simulink model "sys_1_statespace"  (R2017a)
settings: Solver=VariableStepAuto  StartTime=0.0  StopTime=25  FixedStep=0.02  RelTol=1e-3
values from neighbouring files (symbols this model uses):
  A = [0 1 0 0;-k/j2 -b/j2 k/j2 b/j2;0 0 0 01;k/j1 b/j1 -k/j1 -b/j1]    [sys1.m]
  A3 = [0 1 0 0;-k/j2 -b/j2 k/j2 b/j2;0 0 0 01;k/j1 b/j1 -k/j1 -b/j1]    [sys1.m]
  B = [b -b;-b b]    [dynamic_using_Nemark_controller.m]    (also in sys1.m = [0;0;0;1/j1])
  B3 = [0;0;0;1/j1]    [sys1.m]
  C = [1 0 0 0]    [sys1.m]
  C3 = [0 0 1 0;1 0 0 0]    [sys1.m]
  D = zeros(1,1)    [sys1.m]
  D3 = zeros(2,1)    [sys1.m]
undefined symbols (not defined in the file or in its folder): Ad, Bd, Cd, Dd
libraries: simulink x10
settings Model: Creator=ASUS  LastModifiedBy=ASUS

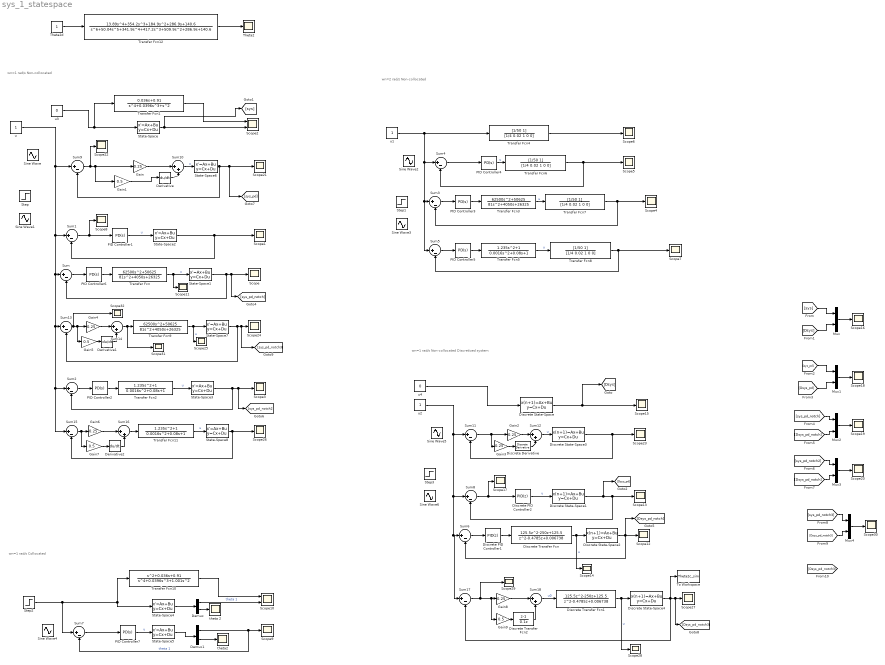
== system sys_1_statespace ==
  note: wn=1 rad/s Non-collocated
  note: wn=2 rad/s Non-collocated
  note: wn=1 rad/s Collocated
  note: wn=1 rad/s Non-collocated
      | Discretized system
  Demux : Demux  Outputs=2
  Demux1 : Demux  Outputs=2
  Derivative : Derivative
  Derivative1 : Derivative
  Derivative2 : Derivative
  Discrete Transfer Fcn : DiscreteTransferFcn  Numerator=[125.5 -250 125.5]  Denominator=[1 -0.4785 0.006738]  SampleTime=0.1
  Discrete Transfer Fcn1 : DiscreteTransferFcn  Numerator=[125.5 -250 125.5]  Denominator=[1 -0.4785 0.006738]  SampleTime=0.1
  Discrete Transfer Fcn2 : DiscreteTransferFcn  Numerator=[1 -1]  Denominator=[0.1 0]  SampleTime=0.1
  Discrete Derivative : simulink/Discrete/Discrete Derivative  gainval=1.0  ICPrevScaledInput=0.0  OutMin=[]  OutMax=[]  OutDataType=fixdt(1, 16)  OutScaling=2^-10  DoSatur=off
  Discrete PID Controller1 : simulink/Continuous/PID Controller  Controller=PID  TimeDomain=Discrete-time  SampleTime=0.1  IntegratorMethod=Forward Euler  FilterMethod=Forward Euler  Form=Parallel  UseFilter=on  ControllerParametersSource=internal  P=0.25  I=0  D=0.5  N=1  InitialConditionSource=internal  InitialConditionForIntegrator=0  InitialConditionForFilter=0  ExternalReset=none  LimitOutput=off  UpperSaturationLimit=inf  LowerSaturationLimit=-inf  LinearizeAsGain=off  AntiWindupMode=none  Kb=1  TrackingMode=off  Kt=1  PParamMin=[]  PParamMax=[]  IParamMin=[]  IParamMax=[]  DParamMin=[]  DParamMax=[]  NParamMin=[]  NParamMax=[]  KbParamMin=[]  KbParamMax=[]  KtParamMin=[]  KtParamMax=[]  POutMin=[]  POutMax=[]  IOutMin=[]  IOutMax=[]  DOutMin=[]  DOutMax=[]  NOutMin=[]  NOutMax=[]  KbOutMin=[]  KbOutMax=[]  KtOutMin=[]  KtOutMax=[]  IntegratorOutMin=[]  IntegratorOutMax=[]  FilterOutMin=[]  FilterOutMax=[]  SumOutMin=[]  SumOutMax=[]  SumI1OutMin=[]  SumI1OutMax=[]  SumI2OutMin=[]  SumI2OutMax=[]  SumI3OutMin=[]  SumI3OutMax=[]  SumDOutMin=[]  SumDOutMax=[]  SaturationOutMin=[]  SaturationOutMax=[]  IntegratorContinuousStateAttributes=''  IntegratorStateMustResolveToSignalObject=off  IntegratorRTWStateStorageClass=Auto  FilterContinuousStateAttributes=''  FilterStateMustResolveToSignalObject=off  FilterRTWStateStorageClass=Auto  DifferentiatorICPrevScaledInput=0  DifferentiatorOutMin=[]  DifferentiatorOutMax=[]  InitialConditionSetting=State (most efficient)
  Discrete PID Controller2 : simulink/Continuous/PID Controller  Controller=PID  TimeDomain=Discrete-time  SampleTime=0.10  IntegratorMethod=Forward Euler  FilterMethod=Forward Euler  Form=Parallel  UseFilter=on  ControllerParametersSource=internal  P=0.25  I=0  D=0.5  N=1  InitialConditionSource=internal  InitialConditionForIntegrator=0  InitialConditionForFilter=0  ExternalReset=none  LimitOutput=off  UpperSaturationLimit=inf  LowerSaturationLimit=-inf  LinearizeAsGain=off  AntiWindupMode=none  Kb=1  TrackingMode=off  Kt=1  PParamMin=[]  PParamMax=[]  IParamMin=[]  IParamMax=[]  DParamMin=[]  DParamMax=[]  NParamMin=[]  NParamMax=[]  KbParamMin=[]  KbParamMax=[]  KtParamMin=[]  KtParamMax=[]  POutMin=[]  POutMax=[]  IOutMin=[]  IOutMax=[]  DOutMin=[]  DOutMax=[]  NOutMin=[]  NOutMax=[]  KbOutMin=[]  KbOutMax=[]  KtOutMin=[]  KtOutMax=[]  IntegratorOutMin=[]  IntegratorOutMax=[]  FilterOutMin=[]  FilterOutMax=[]  SumOutMin=[]  SumOutMax=[]  SumI1OutMin=[]  SumI1OutMax=[]  SumI2OutMin=[]  SumI2OutMax=[]  SumI3OutMin=[]  SumI3OutMax=[]  SumDOutMin=[]  SumDOutMax=[]  SaturationOutMin=[]  SaturationOutMax=[]  IntegratorContinuousStateAttributes=''  IntegratorStateMustResolveToSignalObject=off  IntegratorRTWStateStorageClass=Auto  FilterContinuousStateAttributes=''  FilterStateMustResolveToSignalObject=off  FilterRTWStateStorageClass=Auto  DifferentiatorICPrevScaledInput=0  DifferentiatorOutMin=[]  DifferentiatorOutMax=[]  InitialConditionSetting=State (most efficient)
  Discrete State-Space{,1..4} (5 alike) : DiscreteStateSpace  A=Ad  B=Bd  C=Cd  D=Dd  X0=[0.2 0 0 0]  SampleTime=0.1
  Gain{,2..4,6,8} (6 alike) : Gain  Gain=0.25
  Gain{1,5,7,9} (4 alike) : Gain  Gain=0.5
  Mux{,1..4} (5 alike) : Mux  Inputs=2
  PID Controller{1..3,5,7} (5 alike) : simulink/Continuous/PID Controller  Controller=PD  TimeDomain=Continuous-time  SampleTime=-1  IntegratorMethod=Forward Euler  FilterMethod=Forward Euler  Form=Parallel  UseFilter=on  ControllerParametersSource=internal  P=0.25  I=0  D=0.5  N=100  InitialConditionSource=internal  InitialConditionForIntegrator=0  InitialConditionForFilter=0  ExternalReset=none  LimitOutput=off  UpperSaturationLimit=inf  LowerSaturationLimit=-inf  LinearizeAsGain=on  AntiWindupMode=none  Kb=1  TrackingMode=off  Kt=1  PParamMin=[]  PParamMax=[]  IParamMin=[]  IParamMax=[]  DParamMin=[]  DParamMax=[]  NParamMin=[]  NParamMax=[]  KbParamMin=[]  KbParamMax=[]  KtParamMin=[]  KtParamMax=[]  POutMin=[]  POutMax=[]  IOutMin=[]  IOutMax=[]  DOutMin=[]  DOutMax=[]  NOutMin=[]  NOutMax=[]  KbOutMin=[]  KbOutMax=[]  KtOutMin=[]  KtOutMax=[]  IntegratorOutMin=[]  IntegratorOutMax=[]  FilterOutMin=[]  FilterOutMax=[]  SumOutMin=[]  SumOutMax=[]  SumI1OutMin=[]  SumI1OutMax=[]  SumI2OutMin=[]  SumI2OutMax=[]  SumI3OutMin=[]  SumI3OutMax=[]  SumDOutMin=[]  SumDOutMax=[]  SaturationOutMin=[]  SaturationOutMax=[]  IntegratorContinuousStateAttributes=''  IntegratorStateMustResolveToSignalObject=off  IntegratorRTWStateStorageClass=Auto  FilterContinuousStateAttributes=''  FilterStateMustResolveToSignalObject=off  FilterRTWStateStorageClass=Auto  DifferentiatorICPrevScaledInput=0  DifferentiatorOutMin=[]  DifferentiatorOutMax=[]  InitialConditionSetting=State (most efficient)
  PID Controller4 : simulink/Continuous/PID Controller  Controller=PD  TimeDomain=Continuous-time  SampleTime=-1  IntegratorMethod=Forward Euler  FilterMethod=Forward Euler  Form=Parallel  UseFilter=on  ControllerParametersSource=internal  P=0.001  I=0  D=0.03  N=100  InitialConditionSource=internal  InitialConditionForIntegrator=0  InitialConditionForFilter=0  ExternalReset=none  LimitOutput=off  UpperSaturationLimit=inf  LowerSaturationLimit=-inf  LinearizeAsGain=on  AntiWindupMode=none  Kb=1  TrackingMode=off  Kt=1  PParamMin=[]  PParamMax=[]  IParamMin=[]  IParamMax=[]  DParamMin=[]  DParamMax=[]  NParamMin=[]  NParamMax=[]  KbParamMin=[]  KbParamMax=[]  KtParamMin=[]  KtParamMax=[]  POutMin=[]  POutMax=[]  IOutMin=[]  IOutMax=[]  DOutMin=[]  DOutMax=[]  NOutMin=[]  NOutMax=[]  KbOutMin=[]  KbOutMax=[]  KtOutMin=[]  KtOutMax=[]  IntegratorOutMin=[]  IntegratorOutMax=[]  FilterOutMin=[]  FilterOutMax=[]  SumOutMin=[]  SumOutMax=[]  SumI1OutMin=[]  SumI1OutMax=[]  SumI2OutMin=[]  SumI2OutMax=[]  SumI3OutMin=[]  SumI3OutMax=[]  SumDOutMin=[]  SumDOutMax=[]  SaturationOutMin=[]  SaturationOutMax=[]  IntegratorContinuousStateAttributes=''  IntegratorStateMustResolveToSignalObject=off  IntegratorRTWStateStorageClass=Auto  FilterContinuousStateAttributes=''  FilterStateMustResolveToSignalObject=off  FilterRTWStateStorageClass=Auto  DifferentiatorICPrevScaledInput=0  DifferentiatorOutMin=[]  DifferentiatorOutMax=[]  InitialConditionSetting=State (most efficient)
  PID Controller6 : simulink/Continuous/PID Controller  Controller=PD  TimeDomain=Continuous-time  SampleTime=-1  IntegratorMethod=Forward Euler  FilterMethod=Forward Euler  Form=Parallel  UseFilter=on  ControllerParametersSource=internal  P=0.25  I=0  D=0.5  N=1  InitialConditionSource=internal  InitialConditionForIntegrator=0  InitialConditionForFilter=0  ExternalReset=none  LimitOutput=off  UpperSaturationLimit=inf  LowerSaturationLimit=-inf  LinearizeAsGain=on  AntiWindupMode=none  Kb=1  TrackingMode=off  Kt=1  PParamMin=[]  PParamMax=[]  IParamMin=[]  IParamMax=[]  DParamMin=[]  DParamMax=[]  NParamMin=[]  NParamMax=[]  KbParamMin=[]  KbParamMax=[]  KtParamMin=[]  KtParamMax=[]  POutMin=[]  POutMax=[]  IOutMin=[]  IOutMax=[]  DOutMin=[]  DOutMax=[]  NOutMin=[]  NOutMax=[]  KbOutMin=[]  KbOutMax=[]  KtOutMin=[]  KtOutMax=[]  IntegratorOutMin=[]  IntegratorOutMax=[]  FilterOutMin=[]  FilterOutMax=[]  SumOutMin=[]  SumOutMax=[]  SumI1OutMin=[]  SumI1OutMax=[]  SumI2OutMin=[]  SumI2OutMax=[]  SumI3OutMin=[]  SumI3OutMax=[]  SumDOutMin=[]  SumDOutMax=[]  SaturationOutMin=[]  SaturationOutMax=[]  IntegratorContinuousStateAttributes=''  IntegratorStateMustResolveToSignalObject=off  IntegratorRTWStateStorageClass=Auto  FilterContinuousStateAttributes=''  FilterStateMustResolveToSignalObject=off  FilterRTWStateStorageClass=Auto  DifferentiatorICPrevScaledInput=0  DifferentiatorOutMin=[]  DifferentiatorOutMax=[]  InitialConditionSetting=State (most efficient)
  Scope{,1,3..9,11..32} (31 alike) : Scope
  Scope10 : Scope  NumInputPorts=2
  Scope2 : Scope  NumInputPorts=2
  Sine Wave{,2,4..5} (4 alike) : Sin  Frequency=3  SampleTime=0
  Sine Wave1 : Sin  SampleTime=0
  Sine Wave3 : Sin  SampleTime=0
  Sine Wave6 : Sin  SampleTime=0
  State-Space{,1..3,6..8} (7 alike) : StateSpace  A=A  B=B  C=C  D=D  X0=[0.2 0 0 0]
  State-Space4 : StateSpace  A=A3  B=B3  C=C3  D=D3  X0=0
  State-Space5 : StateSpace  A=A3  B=B3  C=C3  D=D3  X0=0
  Step{,1..3} (4 alike) : Step  SampleTime=0
  Sum{,1..9,11,13,15,17} (14 alike) : Sum  Inputs=|+-
  Sum{10,12,14,16,18} (5 alike) : Sum  Inputs=|++
  Theta2 : Scope
  Theta2d : Constant
  To Workspace : ToWorkspace  VariableName=Theta2c_sim  SaveFormat=Timeseries  SampleTime=0.1
  Transfer Fcn : TransferFcn  Numerator=[62500 0 50625]  Denominator=[81 4050 26325]
  Transfer Fcn1 : TransferFcn  Numerator=[0.036 0.91]  Denominator=[1 0.0396 1 0 0]
  Transfer Fcn10 : TransferFcn  Numerator=[1 0.036 0.91]  Denominator=[1 0.0396 1.001 0 0]
  Transfer Fcn11 : TransferFcn  Numerator=[1.235 0 1]  Denominator=[0.0016 0.08 1]
  Transfer Fcn12 : TransferFcn  Numerator=[13.89 354.2 184.9 286.9 140.6]  Denominator=[1 50.04 341.9 417.2 509.9 286.9 140.6]
  Transfer Fcn2 : TransferFcn  Numerator=[1.235 0 1]  Denominator=[0.0016 0.08 1]
  Transfer Fcn3 : TransferFcn  Numerator=[62500 0 50625]  Denominator=[81 4050 26325]
  Transfer Fcn{4,6..8} (4 alike) : TransferFcn  Numerator=[1/50 1]  Denominator=[1/4 0.02 1 0 0]
  Transfer Fcn5 : TransferFcn  Numerator=[1.235 0 1]  Denominator=[0.0016 0.08 1]
  Transfer Fcn9 : TransferFcn  Numerator=[62500 0 50625]  Denominator=[81 4050 26325]
  theta 2 : Scope
  "theta2 " : Scope
  u : Constant
  u1 : Constant
  u2 : Constant
  u3 : Constant  Value=0
  u4 : Constant  Value=0
  wires:
  Transfer Fcn/1 -> Scope11/1, State-Space1/1  "u"
  u/1 -> Sum9/1, Sum1/1, Sum13/1, Sum15/1, Sum2/1, Sum/1
  State-Space1/1 -> [sys_pd_notch], Scope/1, Sum/2
  Sum/1 -> PID Controller6/1
  PID Controller6/1 -> Transfer Fcn/1
  State-Space2/1 -> Scope1/1, Sum1/2
  PID Controller1/1 -> State-Space2/1  "u"
  Transfer Fcn1/1 -> Scope2/1
  State-Space3/1 -> Sum2/2, [sys_pd_notch2], Scope3/1
  PID Controller2/1 -> Transfer Fcn2/1
  Transfer Fcn2/1 -> State-Space3/1  "u"
  Sum2/1 -> PID Controller2/1
  Sum5/1 -> PID Controller5/1
  Sum4/1 -> PID Controller4/1
  Transfer Fcn6/1 -> Scope5/1, Sum4/2
  Transfer Fcn5/1 -> Transfer Fcn8/1  "u"
  PID Controller5/1 -> Transfer Fcn5/1
  Transfer Fcn8/1 -> Scope7/1, Sum5/2
  u1/1 -> Sum4/1, Sum5/1, Sum3/1, Transfer Fcn4/1
  Transfer Fcn7/1 -> Scope4/1, Sum3/2
  PID Controller3/1 -> Transfer Fcn3/1
  Sum3/1 -> PID Controller3/1
  Transfer Fcn3/1 -> Transfer Fcn7/1  "u"
  Transfer Fcn4/1 -> Scope6/1
  PID Controller4/1 -> Transfer Fcn6/1  "u"
  Transfer Fcn10/1 -> Scope10/1
  PID Controller7/1 -> State-Space5/1  "u"
  Sum7/1 -> PID Controller7/1
  Step2/1 -> State-Space4/1, Transfer Fcn10/1, Sum7/1
  State-Space4/1 -> Demux/1
  Demux/1 -> Scope10/2  "theta 1"
  Demux1/1 -> Scope9/1, Sum7/2  "theta 1"
  State-Space5/1 -> Demux1/1
  Demux/2 -> theta 2/1
  Demux1/2 -> "theta2 "/1
  Sum1/1 -> Scope8/1, PID Controller1/1
  Sum8/1 -> Discrete PID Controller2/1, Scope17/1
  Discrete PID Controller2/1 -> Discrete State-Space1/1  "u"
  Discrete State-Space1/1 -> [Dsys_pd], Sum8/2, Scope13/1
  Discrete PID Controller1/1 -> Discrete Transfer Fcn/1
  Sum6/1 -> Discrete PID Controller1/1
  Discrete State-Space2/1 -> [Dsys_pd_notch], Sum6/2, Scope12/1
  Discrete Transfer Fcn/1 -> Scope14/1, Discrete State-Space2/1  "u"
  Discrete State-Space/1 -> [Dsys], Scope15/1
  State-Space/1 -> [sys], Scope2/2
  [Dsys] -> Mux/2
  [sys] -> Mux/1
  Mux/1 -> Scope16/1
  [Dsys_pd] -> Mux1/2
  [sys_pd] -> Mux1/1
  Mux1/1 -> Scope18/1
  Mux2/1 -> Scope19/1
  [sys_pd_notch] -> Mux2/1
  [Dsys_pd_notch] -> Mux2/2
  [sys_pd_notch2] -> Mux3/1
  Mux3/1 -> Scope20/1
  [Dsys_pd_notch] -> Mux3/2
  Sum9/1 -> Gain/1, Gain1/1, Scope22/1
  Sum10/1 -> State-Space6/1  "u"
  Gain1/1 -> Derivative/1
  Gain/1 -> Sum10/1
  Derivative/1 -> Sum10/2
  State-Space6/1 -> [sys_pd], Scope21/1, Sum9/2
  Sum12/1 -> Discrete State-Space3/1  "u"
  Sum11/1 -> Gain3/1, Gain2/1
  u2/1 -> Sum11/1, Sum17/1, Sum6/1, Sum8/1
  Gain3/1 -> Discrete Derivative/1
  Discrete Derivative/1 -> Sum12/2
  Gain2/1 -> Sum12/1
  Discrete State-Space3/1 -> Scope23/1, Sum11/2
  u3/1 -> Transfer Fcn1/1, State-Space/1
  u4/1 -> Discrete State-Space/1
  State-Space7/1 -> Sum13/2, [sys_pd_notch3], Scope24/1
  Transfer Fcn9/1 -> State-Space7/1, Scope25/1  "u"
  Derivative1/1 -> Sum14/2
  Gain4/1 -> Sum14/1
  Gain5/1 -> Derivative1/1
  Sum13/1 -> Scope32/1, Gain5/1, Gain4/1
  Transfer Fcn11/1 -> State-Space8/1  "u"
  Gain6/1 -> Sum16/1
  State-Space8/1 -> Scope26/1, Sum15/2
  Gain7/1 -> Derivative2/1
  Derivative2/1 -> Sum16/2
  Sum16/1 -> Transfer Fcn11/1
  Sum15/1 -> Gain7/1, Gain6/1
  Discrete Transfer Fcn1/1 -> Discrete State-Space4/1, Scope28/1  "u"
  Discrete State-Space4/1 -> To Workspace/1, [Dsys_pd_notch3], Scope27/1, Sum17/2
  Gain8/1 -> Sum18/1
  Discrete Transfer Fcn2/1 -> Sum18/2
  Gain9/1 -> Discrete Transfer Fcn2/1
  Sum17/1 -> Scope29/1, Gain9/1, Gain8/1
  Sum18/1 -> Discrete Transfer Fcn1/1  "u0"
  [Dsys_pd_notch3] -> Mux4/2
  Mux4/1 -> Scope30/1
  [sys_pd_notch3] -> Mux4/1
  Sum14/1 -> Scope31/1, Transfer Fcn9/1
  Theta2d/1 -> Transfer Fcn12/1
  Transfer Fcn12/1 -> Theta2/1
